simulink model "task3"  (R2019b)
settings: Solver=VariableStepAuto  StartTime=0.0  StopTime=inf  RelTol=1e-3
InitFcn:
  | s=77;
  | t=10000;
libraries: hdlsllib x4, commrandsrc3 x1, simulink x1
settings Model: SimulationMode=accelerator  Creator=zb  LastModifiedBy=zb

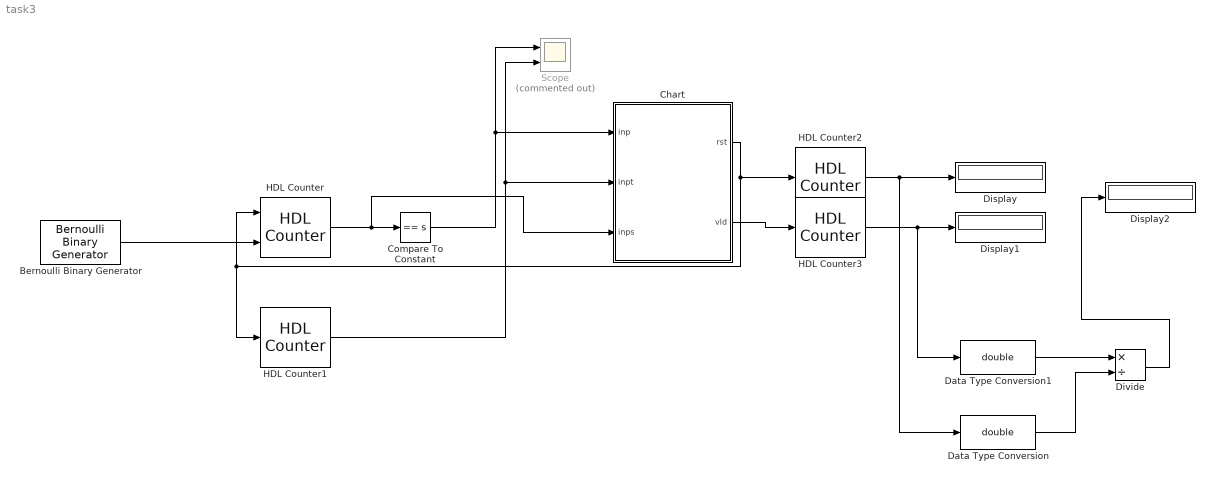
== system task3 ==
  Bernoulli Binary Generator : commrandsrc3/Bernoulli Binary Generator  ProbabilityOfZero=0.99  SeedSource=Auto  Seed=0  SampleTime=1  SamplesPerFrame=1  OutputDataType=boolean  SimulateUsing=Interpreted execution
      settings: SourceProductName=Communications Toolbox
  Chart : Stateflow chart  BlockKeywords=__PRM__SERIALIZED__DATA__:Stateflow Chart,Stateflow Diagram  TreatAsAtomicUnit=on
  Compare To Constant : simulink/Logic and Bit Operations/Compare To Constant  relop===  const=s  OutDataTypeStr=boolean
  Data Type Conversion : DataTypeConversion  OutDataTypeStr=double
  Data Type Conversion1 : DataTypeConversion  OutDataTypeStr=double
  Display : Display
  Display1 : Display
  Display2 : Display
  Divide : Product  Inputs=*/
  HDL Counter : hdlsllib/Sources/HDL Counter  CountType=Count limited  CountInit=0  CountStep=1  CountMax=s  CountFromType=Initial value  CountFrom=0  CountResetPort=on  CountLoadPort=off  CountEnbPort=on  CountDirPort=off  CountDataType=Unsigned  CountWordLen=32  CountFracLen=0  CountSampTime=1
      settings: SourceProductName=Simulink
  HDL Counter1 : hdlsllib/Sources/HDL Counter  CountType=Count limited  CountInit=0  CountStep=1  CountMax=t*5  CountFromType=Initial value  CountFrom=0  CountResetPort=on  CountLoadPort=off  CountEnbPort=off  CountDirPort=off  CountDataType=Unsigned  CountWordLen=32  CountFracLen=0  CountSampTime=1
      settings: SourceProductName=Simulink
  HDL Counter2 : hdlsllib/Sources/HDL Counter  CountType=Free running  CountInit=0  CountStep=1  CountMax=s  CountFromType=Initial value  CountFrom=0  CountResetPort=off  CountLoadPort=off  CountEnbPort=on  CountDirPort=off  CountDataType=Unsigned  CountWordLen=32  CountFracLen=0  CountSampTime=1
      settings: SourceProductName=Simulink
  HDL Counter3 : hdlsllib/Sources/HDL Counter  CountType=Free running  CountInit=0  CountStep=1  CountMax=s  CountFromType=Initial value  CountFrom=0  CountResetPort=off  CountLoadPort=off  CountEnbPort=on  CountDirPort=off  CountDataType=Unsigned  CountWordLen=32  CountFracLen=0  CountSampTime=1
      settings: SourceProductName=Simulink
  Scope : Scope  Commented=on  NumInputPorts=2
  wires:
  Bernoulli Binary Generator/1 -> HDL Counter/2
  HDL Counter/1 -> Chart/3(inps), Compare To Constant/1
  HDL Counter1/1 -> Scope/2, Chart/2(inpt)
  Compare To Constant/1 -> Scope/1, Chart/1(inp)
  Chart/1(rst) -> HDL Counter2/1, HDL Counter/1, HDL Counter1/1
  Chart/2(vld) -> HDL Counter3/1
  HDL Counter2/1 -> Data Type Conversion/1, Display/1
  HDL Counter3/1 -> Data Type Conversion1/1, Display1/1
  Divide/1 -> Display2/1
  Data Type Conversion/1 -> Divide/2
  Data Type Conversion1/1 -> Divide/1

== stateflow chart task3/Chart ==
  state str5
    en:
    s=inps;
    t=inpt;
  state str1
  state str
    en:
    rst = false;
    vld = false;
    s = uint32(0);
    t = uint32(0);
  state str4
    en:
    rst = true;
  state str2
    en:
    vld = true;
    rst = true;
  str5 -> str1 : [inp==false]
  str -> str5 : [inp==true]
  (default) -> str
  str1 -> str4 [order 2]
  str4 -> str
  str1 -> str2 [order 1] : [t<10000]
  str2 -> str
  data: inp input; inpt input; inps input; rst output; vld output; t local; s local
